simulink model "calibrateslx"  (R2019b)
settings: Solver=ode5  StartTime=0.0  StopTime=inf  RelTol=1e-3
libraries: simulink_extras x7, lib_GRM_HIL x2, lib_Serial_PIX x1
settings Model: Creator=guy-m  LastModifiedBy=guy-m
settings RTWCC: Description=Simulink Desktop Real-Time  SystemTargetFile=sldrt.tlc  TemplateMakefile=sldrt.tmf  RTWCompilerOptimization=on
settings CodeAppCC: MaxIdLength=95
settings SimulinkDesktopRealTimeCC: TargetPreCompLibLocation=C:\Program Files\MATLAB\R2019b\toolbox\sldrt\lib\win64  PreserveStateflowLocalDataDimensions=off

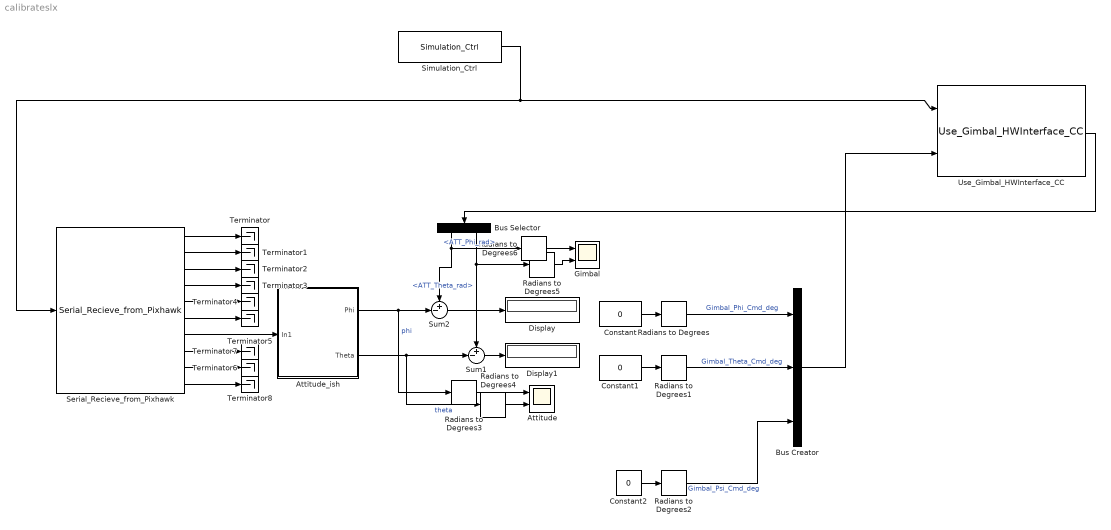
== system calibrateslx ==
  Attitude : Scope  NumInputPorts=2
  Attitude_ish : Subsystem
  Bus Creator : BusCreator  Inputs=3  OutDataTypeStr=Bus: Gimbal_Cmd_Bus
  Bus Selector : BusSelector  OutputSignals=Gimbal_Attitude_Bus.ATT_Euler_Bus.ATT_Phi_rad,Gimbal_Attitude_Bus.ATT_Euler_Bus.ATT_Theta_rad
  Constant : Constant  Value=0
  Constant1 : Constant  Value=0
  Constant2 : Constant  Value=0
  Display : Display
  Display1 : Display
  Gimbal : Scope  NumInputPorts=2
  Radians to Degrees{,1..6} (7 alike) : simulink_extras/Transformations/Radians to Degrees
  Serial_Recieve_from_Pixhawk : lib_Serial_PIX/Serial_Recieve_from_Pixhawk  Serial=HIL_Data.Serial.Pix
      link override Receive_ExternalMode/Packet Input: SampleTime=HIL_Sample_Time  MaxMissedTicks=Serial.Receive.MaxMissedTicks  ShowMissedTicks=off  YieldWhenWaiting=on  DrvName=Standard_Devices/Serial_Port  DrvAddress=3  DrvOptions=[115200 8 0 0 0 0 0 1]  PacketSize=134  DataTypes='134*uint8'  ShowReady=on  ShowError=on  PacketID=1  ByteOrder=1  ShowTimestamp=off
      link override Receive_NormalMode/Serial Receive1: Terminator=<none>  SampleTime=-1
  Simulation_Ctrl : lib_GRM_HIL/Simulation_Ctrl  SystemSampleTime=-1  Latency=0  AutoFrameSizeCalculation=off
  Sum1 : Sum  Inputs=+-|
  Sum2 : Sum  Inputs=+-|
  Terminator{,1..8} (9 alike) : Terminator
  Use_Gimbal_HWInterface_CC : lib_GRM_HIL/Gimbal/Use_Gimbal_HWInterface_CC  SystemSampleTime=-1  VariantControl=VSS_GIMBAL_HWICC  Latency=0  AutoFrameSizeCalculation=off
      link override Communication_FT_HWI_ControlComputer/Receive_from_FTHWICC: SampleTime=HW.SampTime  MaxMissedTicks=100  ShowMissedTicks=off  YieldWhenWaiting=on  DrvName=Standard_Devices/UDP_Protocol  DrvAddress=36864  DrvOptions=[0 36880 49 46 49 46 49 46 49 0 0 0 0 0 0 0 0 0 0 0 0 0 0 0 0 0 0 0 0 0 0 0 0 0 0 0 0 0 0 0 0 0 0 0 0 0 0 0 0 0 0 0 0 0 0 0 0 0 0 0 0 0 0 0 0 0 0 0 0 0 0 0 0 0 0 0 0 0 0 0 0 0 0 0 0 0 0 0 0 0 0 0 0 0 0 0 0 0 0 0 0 0 0 0 0 0 0 0 0 0 0 0 0 0 0 0 0 0 0 0 0 0 0 0 0 0 0 0 0 0 0 0 0 0 0 0 0 0 0 0 0 0 0 0 0 0 0 0 0 0 0 0 0 0 0 0 0 0 0 0 0 0 0 0 0 0 0 0 0 0 0 0 0 0 0 0 0 0 0 0 0 0 0 0 0 0 0 0 0 0 0 0 0 0 0 0 0 0 0 0 0 0 0 0 0 0 0 0 0 0 0 0 0 0 0 0 0 0 0 0 0 0 0 0 0 0 0 0 0 0 0 0 0 0 0 0 0 0 0 0 0 0 0 0 0 0 0 0 0 0 0 0 0 0 0 0]  PacketSize=66  DataTypes={'double','double','double','double','double','double','double','uint16','double'}  ShowReady=on  ShowError=on  PacketID=1  ByteOrder=1  ShowTimestamp=off
      link override Communication_FT_HWI_ControlComputer/Send_to_FTHWICC/Send_to_FTHWICC: SampleTime=1/HIL_Data.Simulation_Ctrl.Com_Ctrl.FT.Com_freq_Hz  MaxMissedTicks=100  ShowMissedTicks=off  YieldWhenWaiting=on  DrvName=Standard_Devices/UDP_Protocol  DrvAddress=36864  DrvOptions=[0 36880 49 57 50 46 49 54 56 46 49 46 49 53 54 0 0 0 0 0 0 0 0 0 0 0 0 0 0 0 0 0 0 0 0 0 0 0 0 0 0 0 0 0 0 0 0 0 0 0 0 0 0 0 0 0 0 0 0 0 0 0 0 0 0 0 0 0 0 0 0 0 0 0 0 0 0 0 0 0 0 0 0 0 0 0 0 0 0 0 0 0 0 0 0 0 0 0 0 0 0 0 0 0 0 0 0 0 0 0 0 0 0 0 0 0 0 0 0 0 0 0 0 0 0 0 0 0 0 0 0 0 0 0 0 0 0 0 0 0 0 0 0 0 0 0 0 0 0 0 0 0 0 0 0 0 0 0 0 0 0 0 0 0 0 0 0 0 0 0 0 0 0 0 0 0 0 0 0 0 0 0 0 0 0 0 0 0 0 0 0 0 0 0 0 0 0 0 0 0 0 0 0 0 0 0 0 0 0 0 0 0 0 0 0 0 0 0 0 0 0 0 0 0 0 0 0 0 0 0 0 0 0 0 0 0 0 0 0 0 0 0 0 0 0 0 0 0 0 0 0 0 0 0 0 0]  PacketSize=52  DataTypes={'boolean','boolean','double','double','uint16','double','double','double','double'}  ShowReady=off  ShowError=off  PacketID=1  ByteOrder=1  InitialValue=[]  FinalValue=[]
  wires:
  Serial_Recieve_from_Pixhawk/1 -> Terminator/1
  Attitude_ish/1(Phi) -> Radians to Degrees3/1, Sum2/2  "phi"
  Use_Gimbal_HWInterface_CC/1 -> Bus Selector/1
  Bus Selector/1 -> Sum2/1, Radians to Degrees6/1  "<ATT_Phi_rad>"
  Simulation_Ctrl/1 -> Serial_Recieve_from_Pixhawk/1, Use_Gimbal_HWInterface_CC/1
  Bus Creator/1 -> Use_Gimbal_HWInterface_CC/2
  Sum1/1 -> Display1/1
  Radians to Degrees/1 -> Bus Creator/1  "Gimbal_Phi_Cmd_deg"
  Attitude_ish/2(Theta) -> Sum1/2, Radians to Degrees4/1  "theta"
  Bus Selector/2 -> Sum1/1, Radians to Degrees5/1  "<ATT_Theta_rad>"
  Serial_Recieve_from_Pixhawk/10 -> Terminator8/1
  Serial_Recieve_from_Pixhawk/2 -> Terminator1/1
  Serial_Recieve_from_Pixhawk/3 -> Terminator2/1
  Serial_Recieve_from_Pixhawk/4 -> Terminator3/1
  Serial_Recieve_from_Pixhawk/5 -> Terminator4/1
  Serial_Recieve_from_Pixhawk/6 -> Terminator5/1
  Serial_Recieve_from_Pixhawk/8 -> Terminator7/1
  Serial_Recieve_from_Pixhawk/7 -> Attitude_ish/1(In1)
  Constant2/1 -> Radians to Degrees2/1
  Radians to Degrees1/1 -> Bus Creator/2  "Gimbal_Theta_Cmd_deg"
  Radians to Degrees2/1 -> Bus Creator/3  "Gimbal_Psi_Cmd_deg"
  Sum2/1 -> Display/1
  Constant/1 -> Radians to Degrees/1
  Serial_Recieve_from_Pixhawk/9 -> Terminator6/1
  Constant1/1 -> Radians to Degrees1/1
  Radians to Degrees3/1 -> Attitude/1
  Radians to Degrees4/1 -> Attitude/2
  Radians to Degrees5/1 -> Gimbal/2
  Radians to Degrees6/1 -> Gimbal/1

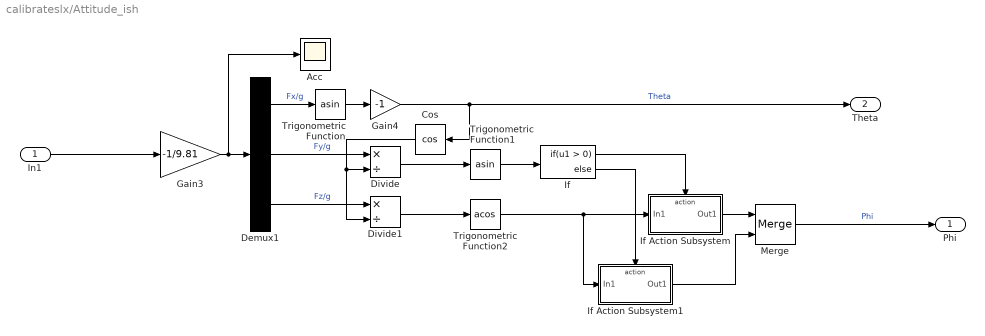
== system calibrateslx/Attitude_ish ==
  In1 : Inport
  Acc : Scope
  Cos : Trigonometry  Operator=cos
  Demux1 : Demux  Outputs=3
  Divide : Product  Inputs=*/
  Divide1 : Product  Inputs=*/
  Gain3 : Gain  Gain=-1/9.81
  Gain4 : Gain  Gain=-1
  If : If
  If Action Subsystem : Subsystem  TreatAsAtomicUnit=on
  If Action Subsystem1 : Subsystem  TreatAsAtomicUnit=on
  Merge : Merge
  Trigonometric Function : Trigonometry  Operator=asin  OutputSignalType=real
  Trigonometric Function1 : Trigonometry  Operator=asin  OutputSignalType=real
  Trigonometric Function2 : Trigonometry  Operator=acos  OutputSignalType=real
  Phi : Outport
  Theta : Outport  Port=2
  wires:
  If/2 -> If Action Subsystem1/Action
  Demux1/1 -> Trigonometric Function/1  "Fx/g"
  Cos/1 -> Divide1/2, Divide/2
  Demux1/2 -> Divide/1  "Fy/g"
  Divide/1 -> Trigonometric Function1/1
  Gain3/1 -> Demux1/1, Acc/1
  Trigonometric Function/1 -> Gain4/1
  Demux1/3 -> Divide1/1  "Fz/g"
  Merge/1 -> Phi/1  "Phi"
  Divide1/1 -> Trigonometric Function2/1
  Gain4/1 -> Theta/1, Cos/1  "Theta"
  Trigonometric Function1/1 -> If/1
  If Action Subsystem/1(Out1) -> Merge/1
  Trigonometric Function2/1 -> If Action Subsystem1/1(In1), If Action Subsystem/1(In1)
  If Action Subsystem1/1(Out1) -> Merge/2
  If/1 -> If Action Subsystem/Action
  In1/1 -> Gain3/1

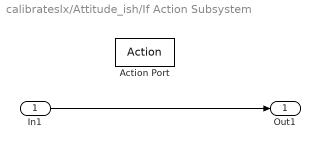
== system calibrateslx/Attitude_ish/If Action Subsystem ==
  In1 : Inport
  Action Port : ActionPort  ActionPortLabel=if(u1 > 0)
  Out1 : Outport
  wires:
  In1/1 -> Out1/1

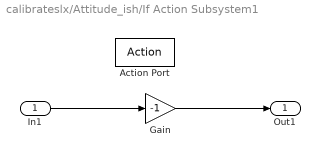
== system calibrateslx/Attitude_ish/If Action Subsystem1 ==
  In1 : Inport
  Action Port : ActionPort  ActionPortLabel=else
  Gain : Gain  Gain=-1
  Out1 : Outport
  wires:
  In1/1 -> Gain/1
  Gain/1 -> Out1/1
